simulink model "L7E2"  (R2020b)
settings: Solver=VariableStepAuto  StartTime=0.0  StopTime=1  MaxStep=1e-6  RelTol=1e-3
libraries: powerlib x16, powerlib_meascontrol x1
settings Model: Creator=Vedant Nath  LastModifiedBy=Vedant Nath
settings DataIOCC: ReturnWorkspaceOutputs=off

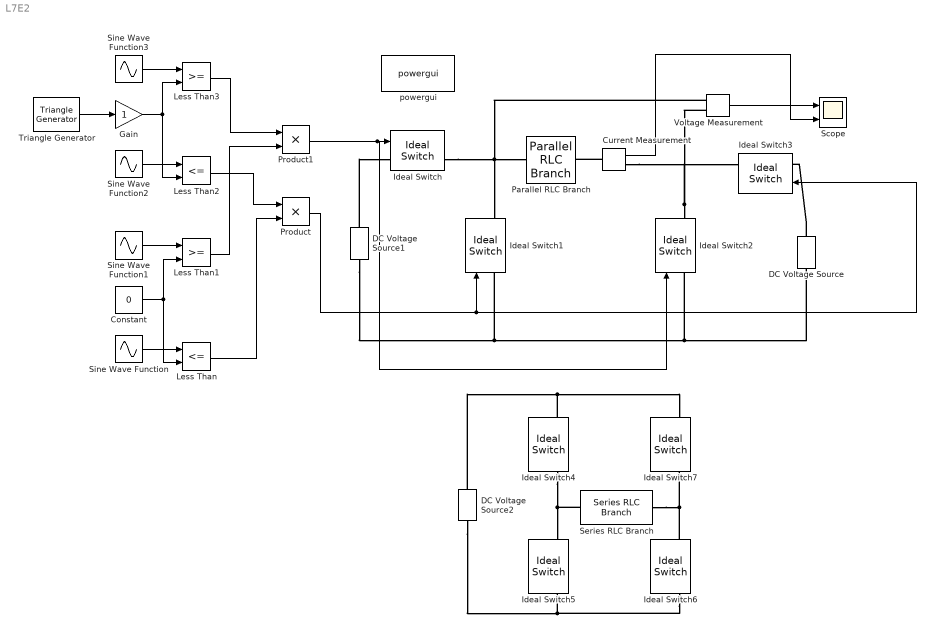
== system L7E2 ==
  Constant : Constant  Value=0
  Current Measurement : powerlib/Measurements/Current Measurement  PhasorSimulation=off  OutputType=Complex  PSBequivalent=0
  DC Voltage Source : powerlib/Electrical Sources/DC Voltage Source  Amplitude=100  Measurements=None
  DC Voltage Source1 : powerlib/Electrical Sources/DC Voltage Source  Amplitude=100  Measurements=None
  DC Voltage Source2 : powerlib/Electrical Sources/DC Voltage Source  Amplitude=100  Measurements=None
  Gain : Gain
  Ideal Switch{,1..7} (8 alike) : powerlib/Power Electronics/Ideal Switch  Ron=0.001  Lon=0  IC=0  Rs=1e5  Cs=inf  Measurements=on
  Less Than : RelationalOperator  Operator=<=  OutDataTypeStr=boolean  RndMeth=Simplest
  Less Than1 : RelationalOperator  OutDataTypeStr=boolean  RndMeth=Simplest
  Less Than2 : RelationalOperator  Operator=<=  OutDataTypeStr=boolean  RndMeth=Simplest
  Less Than3 : RelationalOperator  OutDataTypeStr=boolean  RndMeth=Simplest
  Parallel RLC Branch : powerlib/Elements/Parallel RLC Branch  LConnTagsString=a  RConnTagsString=__new0  BranchType=R  Resistance=10  Inductance=1e-3  SetiL0=off  InitialCurrent=0  Capacitance=1e-6  Setx0=off  InitialVoltage=0  Measurements=None
  Product : Product
  Product1 : Product
  Scope : Scope  NumInputPorts=2
  Series RLC Branch : powerlib/Elements/Series RLC Branch  LConnTagsString=__new0  RConnTagsString=__new0  BranchType=R  Resistance=10  Inductance=1e-3  SetiL0=off  InitialCurrent=0  Capacitance=1e-6  Setx0=off  InitialVoltage=0  Measurements=None
  Sine Wave Function{,1..3} (4 alike) : Sin  Frequency=314.159  SampleTime=0
  Triangle Generator : powerlib_meascontrol/Pulse & Signal Generators/Triangle Generator  Freq=1050  Phase=180  Ts=0
  Voltage Measurement : powerlib/Measurements/Voltage Measurement  PhasorSimulation=off  OutputType=Complex  PSBequivalent=0
  powergui : powerlib/powergui  Priority=1  SimulationMode=Continuous  SampleTime=50e-6  frequency=60  Iterations=50  frequencyindice=0  Pbase=100e6  ErrMax=1e-4  UnitsV=kV  UnitsW=MW  buscounter=0  FunctionMessages=off  echomessages=off  EnableUseOfTLC=off  CurrentSourceSwitches=off  DisableSnubberDevices=off  DisableRonSwitches=off  DisableVfSwitches=off  DisplayEquations=off  AutomaticDiscreteSolvers=off  SolverType=Tustin/Backward Euler (TBE)  Interpol=off  ExternalGateDelay=off  methode=off  Ts=100  x0status=zero  SPID=on  SwTol=0  HookPort=off  NonlinearTolerance=1e-4  nMaxIteration=100  ContinueOnMaxIteration=off  RestoreLinks=warning  ResistiveCurrentMeasurement=off  Frange=[0:2:500]  Ylog=off  Xlog=on  ShowGrid=off  save=off  variable=ZData  structure=ScopeData  ZoomFFT=off  StartTime=0.08  cycles=6  DisplayStyle=1  fundamental=50  FreqAxis=off  MaxFrequency=1500  frequencyindicesteady=1  RmsSteady=1  display=off
  wires:
  Voltage Measurement/1 -> Scope/1
  Sine Wave Function/1 -> Less Than/1
  Sine Wave Function1/1 -> Less Than1/1
  Constant/1 -> Less Than/2, Less Than1/2
  Less Than2/1 -> Product/1
  Less Than1/1 -> Product1/2
  Sine Wave Function2/1 -> Less Than2/1
  Sine Wave Function3/1 -> Less Than3/1
  Gain/1 -> Less Than2/2, Less Than3/2
  Triangle Generator/1 -> Gain/1
  Product1/1 -> Ideal Switch/1, Ideal Switch2/1
  Less Than3/1 -> Product1/1
  Product/1 -> Ideal Switch1/1, Ideal Switch3/1
  Current Measurement/1 -> Scope/2
  Less Than/1 -> Product/2
  connections:
  Ideal Switch/RConn1 -- Parallel RLC Branch/LConn1 -- Voltage Measurement/LConn1 -- Ideal Switch1/RConn1
  Ideal Switch2/RConn1 -- Ideal Switch3/RConn1 -- Current Measurement/RConn1 -- Voltage Measurement/LConn2
  DC Voltage Source1/RConn1 -- Ideal Switch/LConn1
  DC Voltage Source/RConn1 -- Ideal Switch3/LConn1
  DC Voltage Source1/LConn1 -- Ideal Switch1/LConn1 -- Ideal Switch2/LConn1 -- DC Voltage Source/LConn1
  Current Measurement/LConn1 -- Parallel RLC Branch/RConn1
  Ideal Switch6/RConn1 -- Ideal Switch7/LConn1 -- Series RLC Branch/RConn1
  Ideal Switch6/LConn1 -- Ideal Switch5/LConn1 -- DC Voltage Source2/LConn1
  DC Voltage Source2/RConn1 -- Ideal Switch4/LConn1 -- Ideal Switch7/RConn1
  Ideal Switch4/RConn1 -- Series RLC Branch/LConn1 -- Ideal Switch5/RConn1
